simulink model "state_feedback_step_response"  (R2013a)
settings: Solver=ode45  StartTime=0.0  StopTime=30  FixedStep=0.005  RelTol=1e-3
values from neighbouring files (symbols this model uses):
  B1 = a1 + a2*cq2    [mgi_mitsu.m]
undefined symbols (not defined in the file or in its folder): A1, K1, Kp1, qConsigne1, qInitial
settings Model: Creator=Mylene  LastModifiedBy=user
settings DataIOCC: SignalLoggingSaveFormat=ModelDataLogs
settings OptimizationCC: ExpressionDepthLimit=2147483647
settings DebuggingCC: FcnCallInpInsideContextMsg=UseLocalSettings
settings GRTTargetCC: CombineOutputUpdateFcns=off  GRTInterface=on

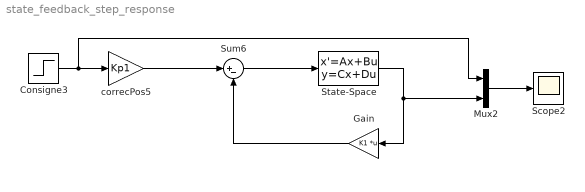
== system state_feedback_step_response ==
  Consigne3 : Step  Before=qInitial  After=qConsigne1  SampleTime=0
  Gain : Gain  Gain=K1  Multiplication=Matrix(K*u)
  Mux2 : Mux  Inputs=2
  Scope2 : Scope
      settings: TimeRange=10  YMin=0  YMax=0.8  SaveName=ScopeData2
  State-Space : StateSpace  A=A1  B=B1  C=eye(2)  D=zeros(2,1)
  Sum6 : Sum  Inputs=|+-
  correcPos5 : Gain  Gain=Kp1
  wires:
  Consigne3/1 -> correcPos5/1, Mux2/1
  Sum6/1 -> State-Space/1
  State-Space/1 -> Gain/1, Mux2/2
  Gain/1 -> Sum6/2
  Mux2/1 -> Scope2/1
  correcPos5/1 -> Sum6/1
